simulink model "unifilar_base"  (Simulink 8.5)
settings: Solver=ode45  StartTime=0.0  StopTime=10.0  RelTol=1e-3
libraries: fm_lib x25
settings Model: Creator=Luis  LastModifiedBy=Luis
settings DataIOCC: SignalLoggingSaveFormat=Dataset
settings OptimizationCC: ExpressionDepthLimit=128
settings DebuggingCC: UnderspecifiedInitializationDetection=Simplified  MergeDetectMultiDrivingBlocksExec=error  FcnCallInpInsideContextMsg=EnableAllAsError  StateNameClashWarn=none
settings GRTTargetCC: CombineOutputUpdateFcns=on  GRTInterface=off

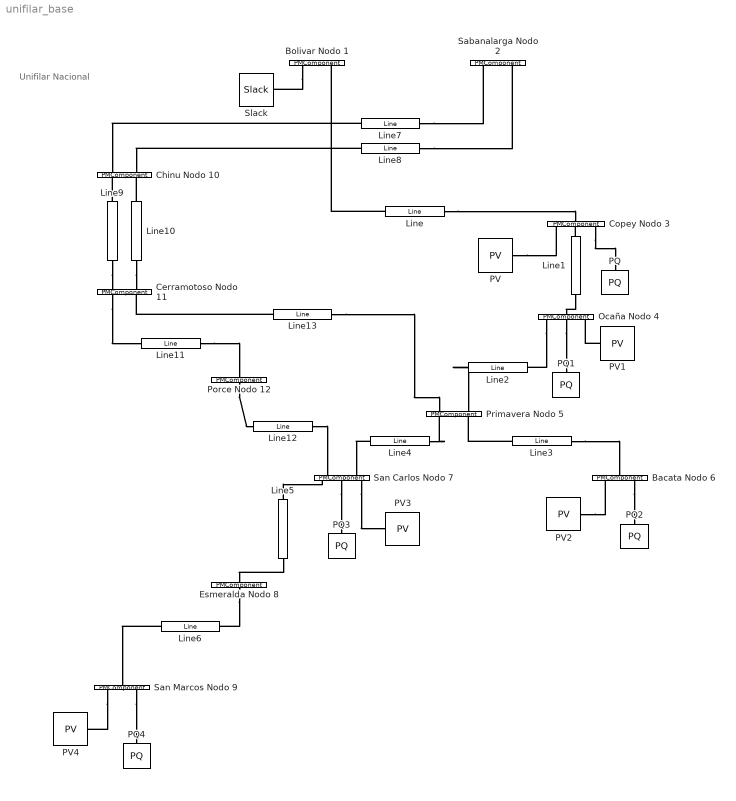
== system unifilar_base ==
  note: Unifilar Nacional
  Bacata Nodo 6 : PMComponent  Tag=PSATblock  Description=Connection  PhysicalDomain=psatdomain  LeftPortType=p1  RightPortType=p1  LConnTagsString=__newl0  RConnTagsString=__newr0|__newr1  mask(Bus){in=1, out=2, p2q=400, p3_4q=[1.00  0.00], p5q=1, p6q=1}
      mask prompts: in "Number of inputs:"; out "Number of outputs:"; p2q "Voltage Rating [kV]"; p3_4q "Voltage initial guess [p.u.  rad]"; p5q "Area number"; p6q "Region number"
      mask help: Bus block.
      mask init:
      | fm_inout
      mask Callback p5q: fm_block
      mask Display: plot([0 1 1 0 0],[0 0 1 1 0])
  Bolivar Nodo 1 : PMComponent  Tag=PSATblock  Description=Connection  PhysicalDomain=psatdomain  LeftPortType=p1  RightPortType=p1  RConnTagsString=__newr0|__newr1  mask(Bus){in=0, out=2, p2q=400, p3_4q=[1.00  0.00], p5q=1, p6q=1}
      mask prompts: in "Number of inputs:"; out "Number of outputs:"; p2q "Voltage Rating [kV]"; p3_4q "Voltage initial guess [p.u.  rad]"; p5q "Area number"; p6q "Region number"
      mask help: Bus block.
      mask init:
      | fm_inout
      mask Callback p5q: fm_block
      mask Display: plot([0 1 1 0 0],[0 0 1 1 0])
  Cerramotoso Nodo 11 : PMComponent  Tag=PSATblock  Description=Connection  PhysicalDomain=psatdomain  LeftPortType=p1  RightPortType=p1  LConnTagsString=__newl0|__newl1  RConnTagsString=__newr0|__newr1  mask(Bus){in=2, out=2, p2q=400, p3_4q=[1.00  0.00], p5q=1, p6q=1}
      mask prompts: in "Number of inputs:"; out "Number of outputs:"; p2q "Voltage Rating [kV]"; p3_4q "Voltage initial guess [p.u.  rad]"; p5q "Area number"; p6q "Region number"
      mask help: Bus block.
      mask init:
      | fm_inout
      mask Callback p5q: fm_block
      mask Display: plot([0 1 1 0 0],[0 0 1 1 0])
  Chinu Nodo 10 : PMComponent  Tag=PSATblock  Description=Connection  PhysicalDomain=psatdomain  LeftPortType=p1  RightPortType=p1  LConnTagsString=__newl0|__newl1  RConnTagsString=__newr0|__newr1  mask(Bus){in=2, out=2, p2q=400, p3_4q=[1.00  0.00], p5q=1, p6q=1}
      mask prompts: in "Number of inputs:"; out "Number of outputs:"; p2q "Voltage Rating [kV]"; p3_4q "Voltage initial guess [p.u.  rad]"; p5q "Area number"; p6q "Region number"
      mask help: Bus block.
      mask init:
      | fm_inout
      mask Callback p5q: fm_block
      mask Display: plot([0 1 1 0 0],[0 0 1 1 0])
  Copey Nodo 3 : PMComponent  Tag=PSATblock  Description=Connection  PhysicalDomain=psatdomain  LeftPortType=p1  RightPortType=p1  LConnTagsString=__newl0  RConnTagsString=__newr0|__newr1|__newr2  mask(Bus){in=1, out=3, p2q=400, p3_4q=[1.00  0.00], p5q=1, p6q=1}
      mask prompts: in "Number of inputs:"; out "Number of outputs:"; p2q "Voltage Rating [kV]"; p3_4q "Voltage initial guess [p.u.  rad]"; p5q "Area number"; p6q "Region number"
      mask help: Bus block.
      mask init:
      | fm_inout
      mask Callback p5q: fm_block
      mask Display: plot([0 1 1 0 0],[0 0 1 1 0])
  Esmeralda Nodo 8 : PMComponent  Tag=PSATblock  Description=Connection  PhysicalDomain=psatdomain  LeftPortType=p1  RightPortType=p1  LConnTagsString=__newl0  RConnTagsString=__newr0  mask(Bus){in=1, out=1, p2q=400, p3_4q=[1.00  0.00], p5q=1, p6q=1}
      mask prompts: in "Number of inputs:"; out "Number of outputs:"; p2q "Voltage Rating [kV]"; p3_4q "Voltage initial guess [p.u.  rad]"; p5q "Area number"; p6q "Region number"
      mask help: Bus block.
      mask init:
      | fm_inout
      mask Callback p5q: fm_block
      mask Display: plot([0 1 1 0 0],[0 0 1 1 0])
  Line{,1..13} (14 alike) : fm_lib/Power Flow/Line  Tag=PSATblock  Description=Power Flow  LConnTagsString=__newl0  RConnTagsString=__newr0  p3_4_5q="[100  400  60]"  p6q=0  p8q=0.01  p9q=0.10  p10q=1e-3  p13_14_15q="[0.0  0.0  0.0]"  p16q=on
  Ocaña Nodo 4 : PMComponent  Tag=PSATblock  Description=Connection  PhysicalDomain=psatdomain  LeftPortType=p1  RightPortType=p1  LConnTagsString=__newl0  RConnTagsString=__newr0|__newr1|__newr2  mask(Bus){in=1, out=3, p2q=400, p3_4q=[1.00  0.00], p5q=1, p6q=1}
      mask prompts: in "Number of inputs:"; out "Number of outputs:"; p2q "Voltage Rating [kV]"; p3_4q "Voltage initial guess [p.u.  rad]"; p5q "Area number"; p6q "Region number"
      mask help: Bus block.
      mask init:
      | fm_inout
      mask Callback p5q: fm_block
      mask Display: plot([0 1 1 0 0],[0 0 1 1 0])
  PQ{,1..4} (5 alike) : fm_lib/Power Flow/PQ  Tag=PSATblock  Description=Power Flow  LConnTagsString=__newl0  p2_3q="[100  400]"  p4_5q="[0.80  0.60]"  p6_7q="[1.2  0.8]"  p8q=on  p9q=on
  PV{,1..4} (5 alike) : fm_lib/Power Flow/PV  Tag=PSATblock  Description=Power Flow  RConnTagsString=__newr0  p2_3q="[100  400]"  p4q=0.8  p5q=1.00  p6_7q="[0.8  -0.2]"  p8_9q="[1.1  0.9]"  p10q=1  p11q=on
  Porce Nodo 12 : PMComponent  Tag=PSATblock  Description=Connection  PhysicalDomain=psatdomain  LeftPortType=p1  RightPortType=p1  LConnTagsString=__newl0  RConnTagsString=__newr0  mask(Bus){in=1, out=1, p2q=400, p3_4q=[1.00  0.00], p5q=1, p6q=1}
      mask prompts: in "Number of inputs:"; out "Number of outputs:"; p2q "Voltage Rating [kV]"; p3_4q "Voltage initial guess [p.u.  rad]"; p5q "Area number"; p6q "Region number"
      mask help: Bus block.
      mask init:
      | fm_inout
      mask Callback p5q: fm_block
      mask Display: plot([0 1 1 0 0],[0 0 1 1 0])
  Primavera Nodo 5 : PMComponent  Tag=PSATblock  Description=Connection  PhysicalDomain=psatdomain  LeftPortType=p1  RightPortType=p1  LConnTagsString=__newl0|__newl1  RConnTagsString=__newr0|__newr1  mask(Bus){in=2, out=2, p2q=400, p3_4q=[1.00  0.00], p5q=1, p6q=1}
      mask prompts: in "Number of inputs:"; out "Number of outputs:"; p2q "Voltage Rating [kV]"; p3_4q "Voltage initial guess [p.u.  rad]"; p5q "Area number"; p6q "Region number"
      mask help: Bus block.
      mask init:
      | fm_inout
      mask Callback p5q: fm_block
      mask Display: plot([0 1 1 0 0],[0 0 1 1 0])
  Sabanalarga Nodo 2 : PMComponent  Tag=PSATblock  Description=Connection  PhysicalDomain=psatdomain  LeftPortType=p1  RightPortType=p1  RConnTagsString=__newr0|__newr1  mask(Bus){in=0, out=2, p2q=400, p3_4q=[1.00  0.00], p5q=1, p6q=1}
      mask prompts: in "Number of inputs:"; out "Number of outputs:"; p2q "Voltage Rating [kV]"; p3_4q "Voltage initial guess [p.u.  rad]"; p5q "Area number"; p6q "Region number"
      mask help: Bus block.
      mask init:
      | fm_inout
      mask Callback p5q: fm_block
      mask Display: plot([0 1 1 0 0],[0 0 1 1 0])
  San Carlos Nodo 7 : PMComponent  Tag=PSATblock  Description=Connection  PhysicalDomain=psatdomain  LeftPortType=p1  RightPortType=p1  LConnTagsString=__newl0|__newl1  RConnTagsString=__newr0|__newr1|__newr2  mask(Bus){in=2, out=3, p2q=400, p3_4q=[1.00  0.00], p5q=1, p6q=1}
      mask prompts: in "Number of inputs:"; out "Number of outputs:"; p2q "Voltage Rating [kV]"; p3_4q "Voltage initial guess [p.u.  rad]"; p5q "Area number"; p6q "Region number"
      mask help: Bus block.
      mask init:
      | fm_inout
      mask Callback p5q: fm_block
      mask Display: plot([0 1 1 0 0],[0 0 1 1 0])
  San Marcos Nodo 9 : PMComponent  Tag=PSATblock  Description=Connection  PhysicalDomain=psatdomain  LeftPortType=p1  RightPortType=p1  LConnTagsString=__newl0  RConnTagsString=__newr0|__newr1  mask(Bus){in=1, out=2, p2q=400, p3_4q=[1.00  0.00], p5q=1, p6q=1}
      mask prompts: in "Number of inputs:"; out "Number of outputs:"; p2q "Voltage Rating [kV]"; p3_4q "Voltage initial guess [p.u.  rad]"; p5q "Area number"; p6q "Region number"
      mask help: Bus block.
      mask init:
      | fm_inout
      mask Callback p5q: fm_block
      mask Display: plot([0 1 1 0 0],[0 0 1 1 0])
  Slack : fm_lib/Power Flow/Slack  Tag=PSATblock  Description=Power Flow  RConnTagsString=__newr0  p2_3q="[100  400]"  p4q=1.00  p5q=0.00  p6_7q="[1.5  -1.5]"  p8_9q="[1.1  0.9]"  p10q=0.80  p11q=1  p12q=on  p13q=on
  connections:
  Line/LConn1 -- Bolivar Nodo 1/RConn2
  Line/RConn1 -- Copey Nodo 3/LConn1
  Line1/RConn1 -- Ocaña Nodo 4/LConn1
  Ocaña Nodo 4/RConn1 -- Line2/RConn1
  Line2/LConn1 -- Primavera Nodo 5/LConn2
  Line3/RConn1 -- Bacata Nodo 6/LConn1
  Line5/LConn1 -- San Carlos Nodo 7/RConn1
  Line5/RConn1 -- Esmeralda Nodo 8/LConn1
  Esmeralda Nodo 8/RConn1 -- Line6/RConn1
  Line6/LConn1 -- San Marcos Nodo 9/LConn1
  Line7/LConn1 -- Chinu Nodo 10/LConn1
  Line7/RConn1 -- Sabanalarga Nodo 2/RConn1
  Line8/LConn1 -- Chinu Nodo 10/LConn2
  Line8/RConn1 -- Sabanalarga Nodo 2/RConn2
  Line9/LConn1 -- Chinu Nodo 10/RConn1
  Line9/RConn1 -- Cerramotoso Nodo 11/LConn1
  Cerramotoso Nodo 11/RConn1 -- Line11/LConn1
  Line11/RConn1 -- Porce Nodo 12/LConn1
  Porce Nodo 12/RConn1 -- Line12/LConn1
  Line12/RConn1 -- San Carlos Nodo 7/LConn1
  Line13/LConn1 -- Cerramotoso Nodo 11/RConn2
  Line13/RConn1 -- Primavera Nodo 5/LConn1
  PV/RConn1 -- Copey Nodo 3/RConn1
  Copey Nodo 3/RConn3 -- PQ/LConn1
  Ocaña Nodo 4/RConn2 -- PQ1/LConn1
  PV1/RConn1 -- Ocaña Nodo 4/RConn3
  Bacata Nodo 6/RConn2 -- PQ2/LConn1
  PV2/RConn1 -- Bacata Nodo 6/RConn1
  San Carlos Nodo 7/RConn2 -- PQ3/LConn1
  San Carlos Nodo 7/RConn3 -- PV3/RConn1
  San Marcos Nodo 9/RConn1 -- PV4/RConn1
  San Marcos Nodo 9/RConn2 -- PQ4/LConn1
  Bolivar Nodo 1/RConn1 -- Slack/RConn1
  Line3/LConn1 -- Primavera Nodo 5/RConn2
  Line1/LConn1 -- Copey Nodo 3/RConn2
  Line4/RConn1 -- Primavera Nodo 5/RConn1
  Line4/LConn1 -- San Carlos Nodo 7/LConn2
  Line10/LConn1 -- Chinu Nodo 10/RConn2
  Line10/RConn1 -- Cerramotoso Nodo 11/LConn2
